simulink model "loadflow"  (R2024a)
settings: Solver=FixedStepAuto  StartTime=0.0  StopTime=15  FixedStep=1e-6  RelTol=1e-3
values from neighbouring files (symbols this model uses):
  D_g1 = 5    [script.m]
  D_g2 = 5    [script.m]
  Elf_g1 = 1.06    [script.m]
  Elf_g2 = 1.15    [script.m]
  fg = 50    [main_v2gg2v.m]    (also in script.m)
  H_g1 = 4    [script.m]
  H_g2 = 1.8    [script.m]
  pairPoles_g1 = 2    [script.m]
  pairPoles_g2 = 3    [script.m]
  Pmlf_g1 = 0.84    [script.m]
  Pmlf_g2 = 0.82    [script.m]
  R_g1 = 0.015    [script.m]
  R_g2 = 0.02    [script.m]
  Rdroop_g1 = 0.05    [script.m]
  Rdroop_g2 = 0.06    [script.m]
  Snom_g1 = 7e6    (= 7000000)    [script.m]
  Snom_g2 = 5e6    (= 5000000)    [script.m]
  Tg_g1 = 0.4    [script.m]
  Tg_g2 = 0.25    [script.m]
  Vac_grid = Vbase    (= 345000)    [script.m]
  X_g1 = 0.3    [script.m]
  X_g2 = 0.35    [script.m]
  Xline_12 = 7/6    (= 1.16666666667)    [script.m]
  Xline_13 = 8/6    (= 1.33333333333)    [script.m]
  Xline_23 = 4/6    (= 0.666666666667)    [script.m]
  Zbase = Vbase^2/Sbase    (= 119025)    [main_v2gg2v.m]    (also in script.m)
libraries: spsThreePhaseVIMeasurementLib x3, spsThreePhaseSeriesRLCBranchLib x3, spsThreePhaseParallelRLCLoadLib x3, eeGeneralControl x2, spsRMSLib x2, spsSimplifiedSynchronousMachinepuUnitsLib x2, spsThreePhaseSourceLib x1, spspowerguiLib x1
settings Model: Creator=hp  LastModifiedBy=hp
settings DebuggingCC: AlgebraicLoopMsg=error  ArtificialAlgebraicLoopMsg=error  BlockPriorityViolationMsg=error  SolverPrmCheckMsg=warning  StateNameClashWarn=warning  OperatingPointInterfaceChecksumMismatchMsg=error
settings HardwareCC: ProdHWDeviceType=AMD->x86-64 (Windows64)
settings DiagnosticsConfigSet: SimMechanicsInvalidVisualProperty=error  SimMechanicsCrossSectionNullEdge=error  SimMechanicsUnconnectedFramePorts=error  SimMechanicsUnconnectedGeometryPorts=error  SimMechanicsRedundantBlock=error  SimMechanicsConflictingReferenceFrames=error  SimMechanicsUnsatisfiedHighPriorityTargets=error

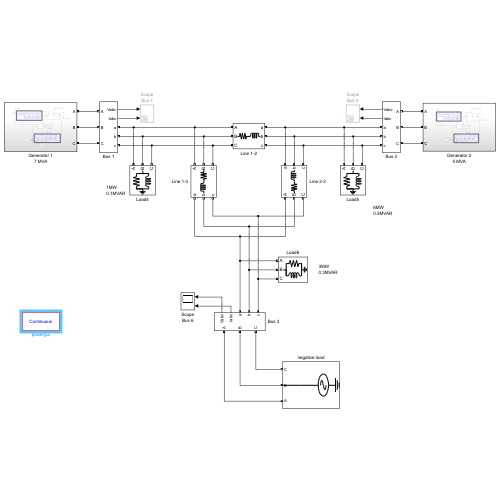
[thumbnail: Simulink's stored preview of the top-level diagram]
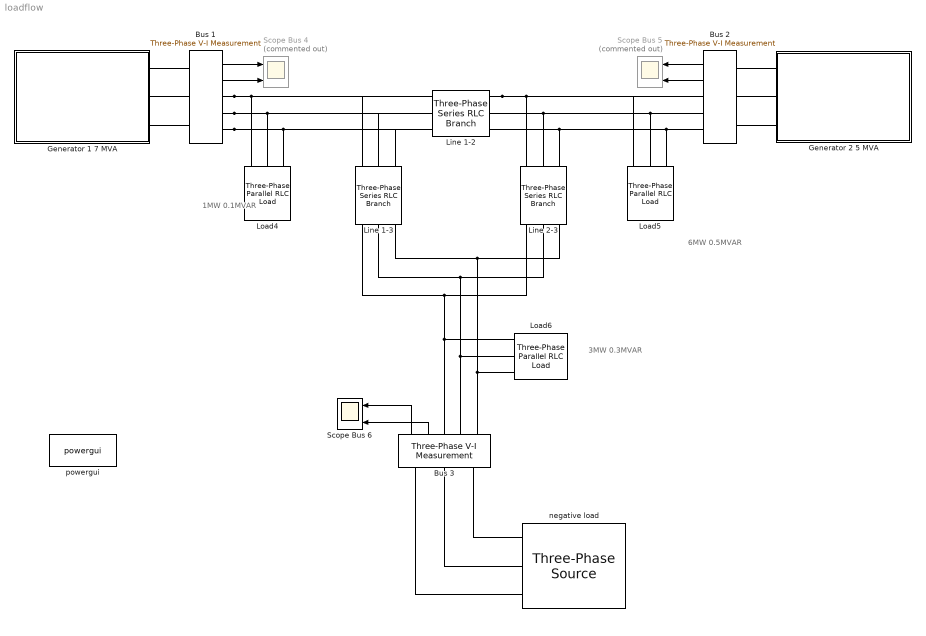
== system loadflow ==
  note: 6MW
      | 0.5MVAR
  note: 3MW
      | 0.3MVAR
  note: 1MW
      | 0.1MVAR
  Bus 1 : spsThreePhaseVIMeasurementLib/Three-Phase V-I Measurement  VoltageMeasurement=phase-to-phase  SetLabelV=off  LabelV=Vabc  Vpu=off  VpuLL=off  CurrentMeasurement=yes  SetLabelI=off  LabelI=Iabc  Ipu=off  Pbase=100e6  Vbase=13.8e3  OutputType=Complex  PhasorSimulation=off  PSBequivalent=0
  Bus 2 : spsThreePhaseVIMeasurementLib/Three-Phase V-I Measurement  VoltageMeasurement=phase-to-phase  SetLabelV=off  LabelV=Vabc  Vpu=off  VpuLL=off  CurrentMeasurement=yes  SetLabelI=off  LabelI=Iabc  Ipu=off  Pbase=100e6  Vbase=13.8e3  OutputType=Complex  PhasorSimulation=off  PSBequivalent=0
  Bus 3 : spsThreePhaseVIMeasurementLib/Three-Phase V-I Measurement  VoltageMeasurement=phase-to-phase  SetLabelV=off  LabelV=Vabc  Vpu=off  VpuLL=off  CurrentMeasurement=yes  SetLabelI=off  LabelI=Iabc  Ipu=off  Pbase=100e6  Vbase=13.8e3  OutputType=Complex  PhasorSimulation=off  PSBequivalent=0
  Generator 1 7 MVA : Subsystem
  Generator 2 5 MVA : Subsystem
  Line 1-2 : spsThreePhaseSeriesRLCBranchLib/Three-Phase Series RLC Branch  LConnTagsString=A|B|C  RConnTagsString=A|B|C  BranchType=RL  Resistance=50*(Xline_12*Zbase)/(2*pi*fg)  Inductance=(Xline_12*Zbase)/(2*pi*fg)  Capacitance=1e-6  Measurements=None
  Line 1-3 : spsThreePhaseSeriesRLCBranchLib/Three-Phase Series RLC Branch  LConnTagsString=A|B|C  RConnTagsString=A|B|C  BranchType=RL  Resistance=50*(Xline_13*Zbase)/(2*pi*fg)  Inductance=(Xline_13*Zbase)/(2*pi*fg)  Capacitance=1e-6  Measurements=None
  Line 2-3 : spsThreePhaseSeriesRLCBranchLib/Three-Phase Series RLC Branch  LConnTagsString=A|B|C  RConnTagsString=A|B|C  BranchType=RL  Resistance=50*(Xline_23*Zbase)/(2*pi*fg)  Inductance=(Xline_23*Zbase)/(2*pi*fg)  Capacitance=1e-6  Measurements=None
  Load4 : spsThreePhaseParallelRLCLoadLib/Three-Phase Parallel RLC Load  LConnTagsString=A|B|C  Configuration=Y (grounded)  NominalVoltage=(230000)*1  Vabc=[1e3 1e3 1e3]  Vabcp=[1e3 1e3 1e3]  NominalFrequency=50  UnbalancedPower=off  ActivePower=1000000  InductivePower=100000  CapacitivePower=0  Pabc=[10e3 9e3 11e3]  QLabc=[100 90 110]  QCabc=[100 90 110]  Pabcp=[10e3 9e3 11e3]  QLabcp=[100 90 110]  QCabcp=[100 90 110]  Measurements=None  LoadType=constant PQ
  Load5 : spsThreePhaseParallelRLCLoadLib/Three-Phase Parallel RLC Load  LConnTagsString=A|B|C  Configuration=Y (grounded)  NominalVoltage=230e3  Vabc=[1e3 1e3 1e3]  Vabcp=[1e3 1e3 1e3]  NominalFrequency=50  UnbalancedPower=off  ActivePower=6000000  InductivePower=500000  CapacitivePower=0  Pabc=[10e3 9e3 11e3]  QLabc=[100 90 110]  QCabc=[100 90 110]  Pabcp=[10e3 9e3 11e3]  QLabcp=[100 90 110]  QCabcp=[100 90 110]  Measurements=None  LoadType=constant PQ
  Load6 : spsThreePhaseParallelRLCLoadLib/Three-Phase Parallel RLC Load  LConnTagsString=A|B|C  Configuration=Y (grounded)  NominalVoltage=230e3  Vabc=[1e3 1e3 1e3]  Vabcp=[1e3 1e3 1e3]  NominalFrequency=50  UnbalancedPower=off  ActivePower=3000000  InductivePower=300000  CapacitivePower=0  Pabc=[10e3 9e3 11e3]  QLabc=[100 90 110]  QCabc=[100 90 110]  Pabcp=[10e3 9e3 11e3]  QLabcp=[100 90 110]  QCabcp=[100 90 110]  Measurements=None  LoadType=constant PQ
  Scope Bus 4 : Scope  Commented=on  NumInputPorts=2
  Scope Bus 5 : Scope  Commented=on  NumInputPorts=2
  Scope Bus 6 : Scope  NumInputPorts=2
  negative load : spsThreePhaseSourceLib/Three-Phase Source  InternalConnection=Yg  VoltagePhases=off  Voltage=230e3  PhaseAngle=0  Voltage_phases=[25e3 25e3 25e3]/sqrt(3)  PhaseAngles_phases=[0 -120 +120]  Frequency=fg  NonIdealSource=off  SpecifyImpedance=off  Resistance=0.8929  Inductance=16.58e-3  ShortCircuitLevel=100e6  BaseVoltage=25e3  XRratio=7  BusType=PQ  Pref=316500  Qref=-30610  Prefabc=[10e3, 10e3, 10e3]  Qrefabc=[0, 0, 0]  Qmin=-Inf  Qmax=Inf
  powergui : spspowerguiLib/powergui  Priority=1  SimulationMode=Continuous  SampleTime=1e-6  frequency=60  Iterations=200  frequencyindice=50  Pbase=100e6  ErrMax=1e-4  UnitsV=kV  UnitsW=MW  buscounter=2  FunctionMessages=off  echomessages=off  EnableUseOfTLC=on  CurrentSourceSwitches=off  DisableSnubberDevices=off  DisableRonSwitches=off  DisableVfSwitches=off  DisplayEquations=off  AutomaticDiscreteSolvers=off  SolverType=Tustin/Backward Euler (TBE)  Interpol=off  ExternalGateDelay=off  methode=off  Ts=100  x0status=blocks  SPID=on  SwTol=0  HookPort=off  NonlinearTolerance=1e-4  nMaxIteration=100  ContinueOnMaxIteration=off  RestoreLinks=warning  ResistiveCurrentMeasurement=off  Frange=[0:2:500]  Ylog=off  Xlog=on  ShowGrid=off  save=off  variable=ZData  structure=0  ZoomFFT=off  StartTime=0.0  cycles=1  DisplayStyle=1  fundamental=60  FreqAxis=off  MaxFrequency=1000  frequencyindicesteady=1  RmsSteady=1  display=off
  wires:
  Bus 1/2 -> Scope Bus 4/2
  Bus 2/2 -> Scope Bus 5/2
  Bus 3/2 -> Scope Bus 6/2
  Bus 1/1 -> Scope Bus 4/1
  Bus 2/1 -> Scope Bus 5/1
  Bus 3/1 -> Scope Bus 6/1
  connections:
  Line 1-2/RConn1 -- Line 2-3/RConn1 -- Load5/LConn1 -- Bus 2/RConn1
  Load5/LConn2 -- Bus 2/RConn2 -- Line 2-3/RConn2 -- Line 1-2/RConn2
  Line 2-3/LConn2 -- Load6/LConn2 -- Bus 3/RConn2 -- Line 1-3/RConn2
  Line 2-3/LConn1 -- Load6/LConn1 -- Bus 3/RConn1 -- Line 1-3/RConn1
  Bus 1/RConn1 -- Load4/LConn1 -- Line 1-3/LConn1 -- Line 1-2/LConn1
  Bus 1/RConn2 -- Load4/LConn2 -- Line 1-3/LConn2 -- Line 1-2/LConn2
  Line 2-3/LConn3 -- Load6/LConn3 -- Bus 3/RConn3 -- Line 1-3/RConn3
  Bus 1/RConn3 -- Load4/LConn3 -- Line 1-3/LConn3 -- Line 1-2/LConn3
  Load5/LConn3 -- Bus 2/RConn3 -- Line 2-3/RConn3 -- Line 1-2/RConn3
  Bus 1/LConn3 -- Generator 1 7 MVA/RConn3
  Bus 2/LConn1 -- Generator 2 5 MVA/RConn1
  Bus 1/LConn1 -- Generator 1 7 MVA/RConn1
  Bus 2/LConn3 -- Generator 2 5 MVA/RConn3
  Bus 1/LConn2 -- Generator 1 7 MVA/RConn2
  Bus 2/LConn2 -- Generator 2 5 MVA/RConn2
  negative load/RConn3 -- Bus 3/LConn3
  negative load/RConn2 -- Bus 3/LConn2
  negative load/RConn1 -- Bus 3/LConn1

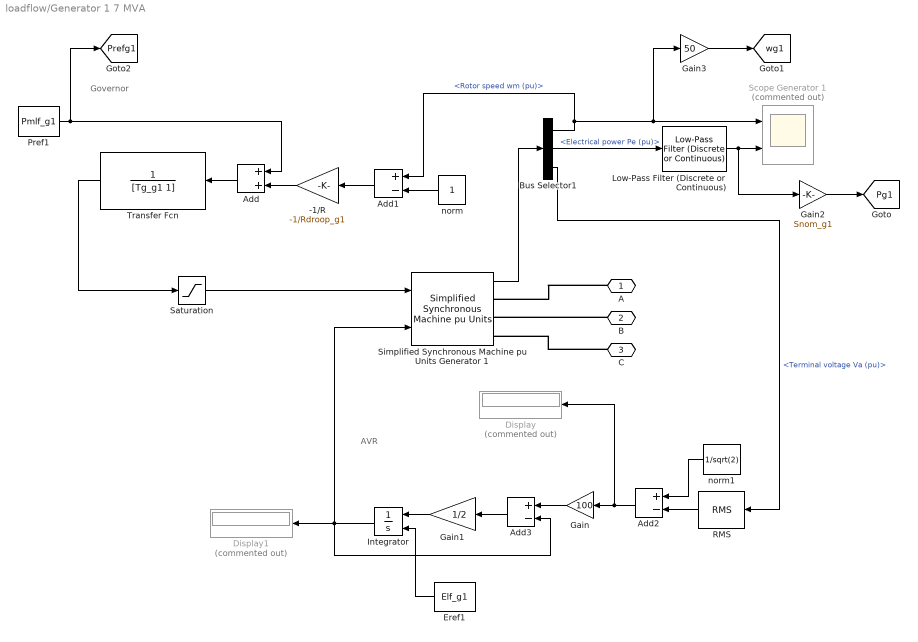
== system loadflow/Generator 1 7 MVA ==
  note: AVR
  note: Governor
  -1/R : Gain  Gain=-1/Rdroop_g1
  Add : Sum
  Add1 : Sum  Inputs=+-
  Add2 : Sum  Inputs=+-
  Add3 : Sum  Inputs=+-
  Bus Selector1 : BusSelector  OutputSignals=Rotor speed wm (pu),Electrical power Pe (pu),Terminal voltage Va (pu)
  Display : Display  Commented=on
  Display1 : Display  Commented=on
  Eref1 : Constant  Value=Elf_g1  SampleTime=1e-6
  Gain : Gain  Gain=100
  Gain1 : Gain  Gain=1/2
  Gain2 : Gain  Gain=Snom_g1
  Gain3 : Gain  Gain=50
  Integrator : Integrator  InitialConditionSource=external  InitialCondition=Elf_g1  LimitOutput=on  UpperSaturationLimit=1.3  LowerSaturationLimit=0.7
  Low-Pass Filter (Discrete or Continuous) : eeGeneralControl/Low-Pass Filter (Discrete or Continuous)  K=1  T=1/(2*pi*15)  B=inf  A=-inf  init_option=Inherited from block input  x0=0  Ts=-1
  Pref1 : Constant  Value=Pmlf_g1  SampleTime=1e-6
  RMS : spsRMSLib/RMS  TrueRMS=on  Freq=50  RMSInit=0.707  Ts=1e-6
  Saturation : Saturate  UpperLimit=1.1  LowerLimit=0.05
  Scope Generator 1 : Scope  Commented=on  NumInputPorts=2
  Simplified Synchronous Machine pu Units Generator 1 : spsSimplifiedSynchronousMachinepuUnitsLib/Simplified Synchronous Machine pu Units  ConnectionType=3-wire Y  MechanicalLoad=Mechanical power Pm  MeasurementBus=off  NominalParameters=[Snom_g1 Vac_grid fg]  Mechanical=[H_g1 D_g1 pairPoles_g1]  InternalRL="[R_g1  X_g1]"  InitialConditions=[0 13.6621 0.836176 0.836176 0.836176 -3.35781 -123.358 116.642]  IterativeDiscreteModel=Trapezoidal non iterative  TsBlock=1e-6  TsPowergui=0  LoadFlowParameters=[1 0 0 0 0]  Units=0  BusType=swing  Pref=6000000  Qref=0  Qmin=-2100000  Qmax=2800000  PLF=0  QLF=0
      settings: LibrarySourceBlock=|
      | sps_lib/Electrical Machines/Simplified Synchronous
      | Machine pu Units
  Transfer Fcn : TransferFcn  Denominator=[Tg_g1 1]
  norm : Constant  SampleTime=1e-6
  norm1 : Constant  Value=1/sqrt(2)  SampleTime=1e-6
  A : PMIOPort  Side=Right
  B : PMIOPort  Port=2  Side=Right
  C : PMIOPort  Port=3  Side=Right
  tag scope: Pg1=global, Prefg1=global, wg1=global
  wires:
  Transfer Fcn/1 -> Saturation/1
  Bus Selector1/1 -> Add1/1, Gain3/1, Scope Generator 1/1  "<Rotor speed wm (pu)>"
  Bus Selector1/2 -> Low-Pass Filter (Discrete or Continuous)/1  "<Electrical power Pe (pu)>"
  Simplified Synchronous Machine pu Units Generator 1/1 -> Bus Selector1/1
  Add/1 -> Transfer Fcn/1
  -1/R/1 -> Add/2
  norm/1 -> Add1/2
  Add1/1 -> -1/R/1
  Saturation/1 -> Simplified Synchronous Machine pu Units Generator 1/1
  Pref1/1 -> [Prefg1], Add/1
  Low-Pass Filter (Discrete or Continuous)/1 -> Gain2/1, Scope Generator 1/2
  Bus Selector1/3 -> RMS/1  "<Terminal voltage Va (pu)>"
  RMS/1 -> Add2/2
  norm1/1 -> Add2/1
  Add2/1 -> Display/1, Gain/1
  Gain/1 -> Add3/1
  Add3/1 -> Gain1/1
  Gain1/1 -> Integrator/1
  Integrator/1 -> Simplified Synchronous Machine pu Units Generator 1/2, Display1/1, Add3/2
  Eref1/1 -> Integrator/2
  Gain2/1 -> [Pg1]
  Gain3/1 -> [wg1]
  connections:
  A/RConn1 -- Simplified Synchronous Machine pu Units Generator 1/RConn1
  C/RConn1 -- Simplified Synchronous Machine pu Units Generator 1/RConn3
  B/RConn1 -- Simplified Synchronous Machine pu Units Generator 1/RConn2

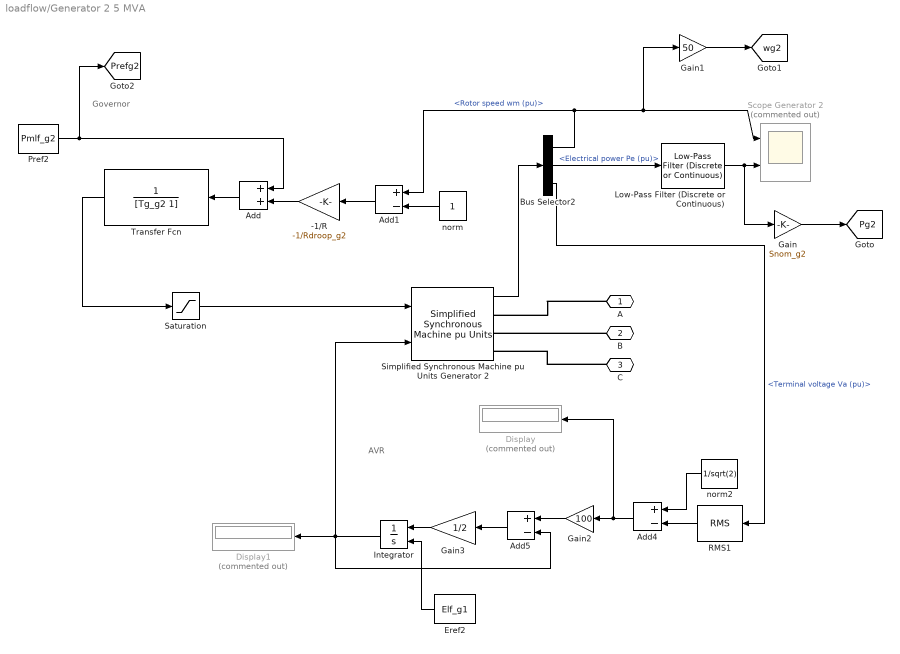
== system loadflow/Generator 2 5 MVA ==
  note: AVR
  note: Governor
  -1/R : Gain  Gain=-1/Rdroop_g2
  Add : Sum
  Add1 : Sum  Inputs=+-
  Add4 : Sum  Inputs=+-
  Add5 : Sum  Inputs=+-
  Bus Selector2 : BusSelector  OutputSignals=Rotor speed wm (pu),Electrical power Pe (pu),Terminal voltage Va (pu)
  Display : Display  Commented=on
  Display1 : Display  Commented=on
  Eref2 : Constant  Value=Elf_g1  SampleTime=1e-6
  Gain : Gain  Gain=Snom_g2
  Gain1 : Gain  Gain=50
  Gain2 : Gain  Gain=100
  Gain3 : Gain  Gain=1/2
  Integrator : Integrator  InitialConditionSource=external  InitialCondition=Elf_g2  LimitOutput=on  UpperSaturationLimit=1.3  LowerSaturationLimit=0.7
  Low-Pass Filter (Discrete or Continuous) : eeGeneralControl/Low-Pass Filter (Discrete or Continuous)  K=1  T=1/(2*pi*15)  B=inf  A=-inf  init_option=Inherited from block input  x0=0  Ts=-1
  Pref2 : Constant  Value=Pmlf_g2  SampleTime=1e-6
  RMS1 : spsRMSLib/RMS  TrueRMS=on  Freq=50  RMSInit=0.707  Ts=1e-6
  Saturation : Saturate  UpperLimit=1.1  LowerLimit=0.05
  Scope Generator 2 : Scope  Commented=on  NumInputPorts=2
  Simplified Synchronous Machine pu Units Generator 2 : spsSimplifiedSynchronousMachinepuUnitsLib/Simplified Synchronous Machine pu Units  ConnectionType=3-wire Y  MechanicalLoad=Mechanical power Pm  MeasurementBus=off  NominalParameters=[Snom_g2 Vac_grid fg]  Mechanical=[H_g2 D_g2 pairPoles_g2]  InternalRL="[R_g2  X_g2]"  InitialConditions=[0 3.78666 0.863133 0.863133 0.863133 -30.7664 -150.766 89.2336]  IterativeDiscreteModel=Trapezoidal non iterative  TsBlock=1e-6  TsPowergui=0  LoadFlowParameters=[1,0,0,0,0]  Units=0  BusType=PV  Pref=4000000  Qref=0  Qmin=-1250000  Qmax=1500000  PLF=0  QLF=0
      settings: LibrarySourceBlock=|
      | sps_lib/Electrical Machines/Simplified Synchronous
      | Machine pu Units
  Transfer Fcn : TransferFcn  Denominator=[Tg_g2 1]
  norm : Constant  SampleTime=1e-6
  norm2 : Constant  Value=1/sqrt(2)  SampleTime=1e-6
  A : PMIOPort  Side=Right
  B : PMIOPort  Port=2  Side=Right
  C : PMIOPort  Port=3  Side=Right
  tag scope: Pg2=global, Prefg2=global, wg2=global
  wires:
  Bus Selector2/1 -> Add1/1, Gain1/1, Scope Generator 2/1  "<Rotor speed wm (pu)>"
  Simplified Synchronous Machine pu Units Generator 2/1 -> Bus Selector2/1
  norm/1 -> Add1/2
  Add1/1 -> -1/R/1
  Add/1 -> Transfer Fcn/1
  -1/R/1 -> Add/2
  Bus Selector2/2 -> Low-Pass Filter (Discrete or Continuous)/1  "<Electrical power Pe (pu)>"
  Transfer Fcn/1 -> Saturation/1
  Saturation/1 -> Simplified Synchronous Machine pu Units Generator 2/1
  Pref2/1 -> [Prefg2], Add/1
  Bus Selector2/3 -> RMS1/1  "<Terminal voltage Va (pu)>"
  norm2/1 -> Add4/1
  RMS1/1 -> Add4/2
  Add4/1 -> Display/1, Gain2/1
  Gain3/1 -> Integrator/1
  Integrator/1 -> Simplified Synchronous Machine pu Units Generator 2/2, Display1/1, Add5/2
  Gain2/1 -> Add5/1
  Add5/1 -> Gain3/1
  Eref2/1 -> Integrator/2
  Low-Pass Filter (Discrete or Continuous)/1 -> Gain/1, Scope Generator 2/2
  Gain/1 -> [Pg2]
  Gain1/1 -> [wg2]
  connections:
  B/RConn1 -- Simplified Synchronous Machine pu Units Generator 2/RConn2
  A/RConn1 -- Simplified Synchronous Machine pu Units Generator 2/RConn1
  C/RConn1 -- Simplified Synchronous Machine pu Units Generator 2/RConn3
